simulink model "gm_combinedTxRx_AXIMM"  (R2017b)
settings: Solver=FixedStepDiscrete  StartTime=0.0  StopTime=10.0  RelTol=1e-3
InitFcn:
  | modelSettings
undefined symbols (not defined in the file or in its folder): coeff, filt, j, RadioSampleRate, VibertiTracebackLength, xPreambleSeq
libraries: hdlmdlgenlib x24, simulink x20, dsphdlfiltering x20, hdlsllib x10, dspsigops x5, commseqgen3 x4, commdigbbndpm3 x3, commcrc2 x2, commcnvcod2 x2, commsource2 x1, dspstat3 x1, dspmlti4 x1
(part 1 of 6)
settings Model: Creator=tcollins  LastModifiedBy=tcollins
settings OptimizationCC: BlockReduction=off  ConditionallyExecuteInputs=off  DefaultParameterBehavior=Inlined
settings DebuggingCC: AlgebraicLoopMsg=error  ArtificialAlgebraicLoopMsg=none  InheritedTsInSrcMsg=none  SingleTaskRateTransMsg=error  ParameterPrecisionLossMsg=none
settings HardwareCC: ProdBitPerPointer=32  ProdBitPerSizeT=32  ProdBitPerPtrDiffT=32  ProdLargestAtomicFloat=None  ProdIntDivRoundTo=Undefined  ProdEndianess=Unspecified  ProdWordSize=32  ProdHWDeviceType=ASIC/FPGA->ASIC/FPGA  ProdEqTarget=off
settings CodeAppCC: StateflowObjectComments=on

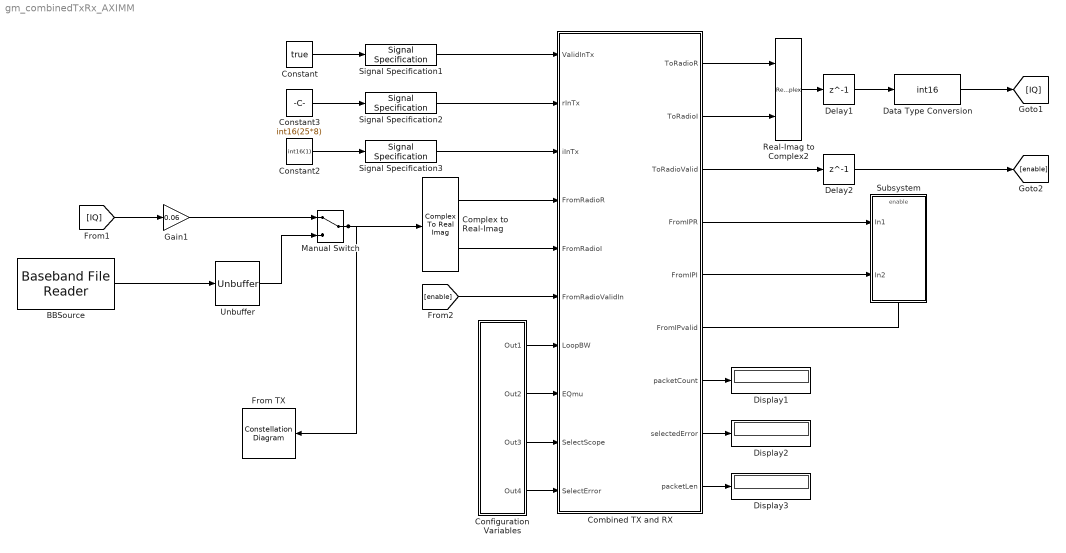
== system gm_combinedTxRx_AXIMM ==
  BBSource : commsource2/Baseband File Reader  Filename=PlutoCaptureQPSK.bb  InheritSampleTimeFromFile=off  SampleTime=100000/(RadioSampleRate)  SamplesPerFrame=100000  CyclicRepetition=off  FileEndOutputPort=off  SimulateUsing=Interpreted execution
      settings: SourceProductName=Communications System Toolbox  SourceProductBaseCode=CM
  Combined TX and RX : Subsystem  TreatAsAtomicUnit=on
  Complex to Real-Imag : ComplexToRealImag
  Configuration Variables : Subsystem
  Constant : Constant  Value=true  SampleTime=-1
  Constant2 : Constant  Value=int16(1)  SampleTime=-1
  Constant3 : Constant  Value=int16(25*8)  SampleTime=-1
  Data Type Conversion : DataTypeConversion  OutDataTypeStr=int16  ConvertRealWorld=Stored Integer (SI)
  Delay1 : Delay  DelayLength=1
  Delay2 : Delay  DelayLength=1
  Display1 : Display
  Display2 : Display
  Display3 : Display
  From TX : ConstellationDiagram
  Gain1 : Gain  Gain=0.06  OutDataTypeStr=int16
  Manual Switch : ManualSwitch
  Real-Imag to Complex2 : RealImagToComplex
  Signal Specification1 : SignalSpecification  OutDataTypeStr=boolean  SampleTime=1/RadioSampleRate
  Signal Specification2 : SignalSpecification  OutDataTypeStr=int16  SampleTime=1/RadioSampleRate
  Signal Specification3 : SignalSpecification  OutDataTypeStr=int16  SampleTime=1/RadioSampleRate
  Subsystem : Subsystem
  Unbuffer : Unbuffer
  wires:
  Configuration Variables/4(Out4) -> Combined TX and RX/10(SelectError)
  Combined TX and RX/9(packetLen) -> Display3/1
  Combined TX and RX/8(selectedError) -> Display2/1
  Combined TX and RX/7(packetCount) -> Display1/1
  Combined TX and RX/6(FromIPvalid) -> Subsystem/Enable
  Combined TX and RX/5(FromIPI) -> Subsystem/2(In2)
  Combined TX and RX/4(FromIPR) -> Subsystem/1(In1)
  Configuration Variables/3(Out3) -> Combined TX and RX/9(SelectScope)
  Configuration Variables/2(Out2) -> Combined TX and RX/8(EQmu)
  Configuration Variables/1(Out1) -> Combined TX and RX/7(LoopBW)
  Real-Imag to Complex2/1 -> Delay1/1
  Combined TX and RX/2(ToRadioI) -> Real-Imag to Complex2/2
  Combined TX and RX/1(ToRadioR) -> Real-Imag to Complex2/1
  Unbuffer/1 -> Manual Switch/2
  Complex to Real-Imag/2 -> Combined TX and RX/5(FromRadioI)
  Complex to Real-Imag/1 -> Combined TX and RX/4(FromRadioR)
  Gain1/1 -> Manual Switch/1
  [IQ] -> Gain1/1
  Signal Specification2/1 -> Combined TX and RX/2(rInTx)
  Manual Switch/1 -> Complex to Real-Imag/1, From TX/1
  Delay2/1 -> [enable]
  Data Type Conversion/1 -> [IQ]
  Delay1/1 -> Data Type Conversion/1
  Combined TX and RX/3(ToRadioValid) -> Delay2/1
  [enable] -> Combined TX and RX/6(FromRadioValidIn)
  Signal Specification3/1 -> Combined TX and RX/3(iInTx)
  Signal Specification1/1 -> Combined TX and RX/1(ValidInTx)
  BBSource/1 -> Unbuffer/1
  Constant/1 -> Signal Specification1/1
  Constant2/1 -> Signal Specification3/1
  Constant3/1 -> Signal Specification2/1

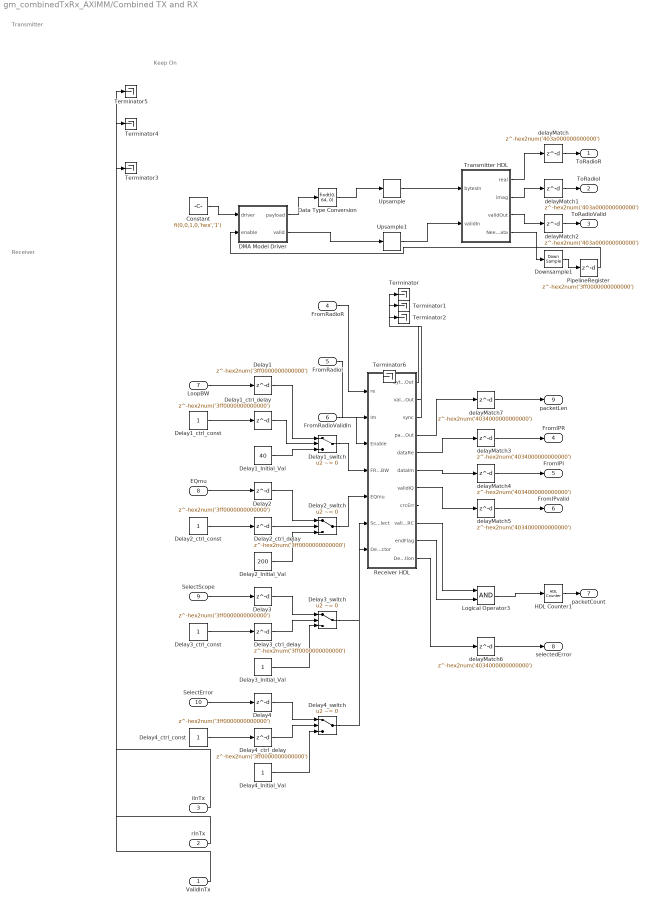
== system gm_combinedTxRx_AXIMM/Combined TX and RX ==
  note: Keep On
  note: Transmitter
  note: Receiver
  ValidInTx : Inport  OutDataTypeStr=boolean  SampleTime=1e-06
  rInTx : Inport  Port=2  OutDataTypeStr=int16  SampleTime=1e-06
  iInTx : Inport  Port=3  OutDataTypeStr=int16  SampleTime=1e-06
  FromRadioR : Inport  Port=4  OutDataTypeStr=int16  PortDimensions=1  SampleTime=1e-06
  FromRadioI : Inport  Port=5  OutDataTypeStr=int16  PortDimensions=1  SampleTime=1e-06
  FromRadioValidIn : Inport  Port=6  OutDataTypeStr=boolean  SampleTime=1e-06
  LoopBW : Inport  Port=7  OutDataTypeStr=int16  SampleTime=1e-06
  EQmu : Inport  Port=8  OutDataTypeStr=int16  SampleTime=1e-06
  SelectScope : Inport  Port=9  OutDataTypeStr=int8  SampleTime=1e-06
  SelectError : Inport  Port=10  OutDataTypeStr=int8  SampleTime=1e-06
  Constant : Constant  Value=fi(0,0,1,0,'hex','1')  OutDataTypeStr=boolean  SampleTime=-1
  DMA Model Driver : Subsystem
  Data Type Conversion : DataTypeConversion  OutDataTypeStr=fixdt(0, 64, 0)  SampleTime=4e-06
  Delay{1..4} (4 alike) : Delay  DelayLength=hex2num('3ff0000000000000')  InitialCondition=0  InputProcessing=Inherited  SampleTime=1e-06
  Delay1_Initial_Val : Constant  Value=40  OutDataTypeStr=int16  SampleTime=-1
  Delay1_ctrl_const : Constant  OutDataTypeStr=boolean  SampleTime=1e-06
  Delay1_ctrl_delay : Delay  DelayLength=hex2num('3ff0000000000000')  InitialCondition=0  InputProcessing=Inherited  SampleTime=1e-06
  Delay1_switch : Switch  Criteria=u2 ~= 0  Threshold=hex2num('0000000000000000')  OutDataTypeStr=int16  SampleTime=1e-06
  Delay2_Initial_Val : Constant  Value=200  OutDataTypeStr=int16  SampleTime=-1
  Delay2_ctrl_const : Constant  OutDataTypeStr=boolean  SampleTime=1e-06
  Delay2_ctrl_delay : Delay  DelayLength=hex2num('3ff0000000000000')  InitialCondition=0  InputProcessing=Inherited  SampleTime=1e-06
  Delay2_switch : Switch  Criteria=u2 ~= 0  Threshold=hex2num('0000000000000000')  OutDataTypeStr=int16  SampleTime=1e-06
  Delay3_Initial_Val : Constant  OutDataTypeStr=int8  SampleTime=-1
  Delay3_ctrl_const : Constant  OutDataTypeStr=boolean  SampleTime=1e-06
  Delay3_ctrl_delay : Delay  DelayLength=hex2num('3ff0000000000000')  InitialCondition=0  InputProcessing=Inherited  SampleTime=1e-06
  Delay3_switch : Switch  Criteria=u2 ~= 0  Threshold=hex2num('0000000000000000')  OutDataTypeStr=int8  SampleTime=1e-06
  Delay4_Initial_Val : Constant  OutDataTypeStr=int8  SampleTime=-1
  Delay4_ctrl_const : Constant  OutDataTypeStr=boolean  SampleTime=1e-06
  Delay4_ctrl_delay : Delay  DelayLength=hex2num('3ff0000000000000')  InitialCondition=0  InputProcessing=Inherited  SampleTime=1e-06
  Delay4_switch : Switch  Criteria=u2 ~= 0  Threshold=hex2num('0000000000000000')  OutDataTypeStr=int8  SampleTime=1e-06
  Downsample1 : DownSample  N=hex2num('4010000000000000')  phase=hex2num('0000000000000000')  RateOptions=Allow multirate processing
  HDL Counter1 : hdlsllib/Sources/HDL Counter  CountType=Count limited  CountInit=hex2num('0000000000000000')  CountStep=hex2num('3ff0000000000000')  CountMax=hex2num('41efffffffe00000')  CountFromType=Initial value  CountFrom=hex2num('0000000000000000')  CountResetPort=off  CountLoadPort=off  CountEnbPort=on  CountDirPort=off  CountDataType=Unsigned  CountWordLen=32  CountFracLen=0  CountSampTime=1e-06
      settings: SourceProductBaseCode=HD
  Logical Operator3 : Logic  AllPortsSameDT=off  OutDataTypeStr=boolean  SampleTime=1e-06
  PipelineRegister : Delay  DelayLength=hex2num('3ff0000000000000')  InitialCondition=0  InputProcessing=Inherited  SampleTime=4e-06
  Receiver HDL : Subsystem
      mask Display:
      | if ispc
      |     d = '\';
      | else
      |     d = '/';
      | end
      | model_path = get_param(bdroot, 'FileName');
      | %info = Simulink.MDLInfo(bdroot)
      | c = strsplit(model_path,d); c = strjoin(c(1:end-2),d);
      | logo = [c,d,'ADI_logo.svg'];
      | %disp(logo);
      | image(logo);
  Terminator{,1..6} (7 alike) : Terminator
  Transmitter HDL : Subsystem
      mask Display:
      | if ispc
      |     d = '\';
      | else
      |     d = '/';
      | end
      | model_path = get_param(bdroot, 'FileName');
      | %info = Simulink.MDLInfo(bdroot)
      | c = strsplit(model_path,d); c = strjoin(c(1:end-2),d);
      | logo = [c,d,'ADI_logo.svg'];
      | %disp(logo);
      | image(logo);
  Upsample : dspsigops/Upsample  N=hex2num('4010000000000000')  phase=hex2num('0000000000000000')  RateOptions=Allow multirate processing  ic=0  mode=Unused parameter value
  Upsample1 : dspsigops/Upsample  N=hex2num('4010000000000000')  phase=hex2num('0000000000000000')  RateOptions=Allow multirate processing  ic=0  mode=Unused parameter value
  delayMatch : Delay  DelayLength=hex2num('403a000000000000')  InitialCondition=0  InputProcessing=Inherited  SampleTime=1e-06
  delayMatch1 : Delay  DelayLength=hex2num('403a000000000000')  InitialCondition=0  InputProcessing=Inherited  SampleTime=1e-06
  delayMatch2 : Delay  DelayLength=hex2num('403a000000000000')  InitialCondition=0  InputProcessing=Inherited  SampleTime=1e-06
  delayMatch{3..7} (5 alike) : Delay  DelayLength=hex2num('4034000000000000')  InitialCondition=0  InputProcessing=Inherited  SampleTime=1e-06
  ToRadioR : Outport
  ToRadioI : Outport  Port=2
  ToRadioValid : Outport  Port=3
  FromIPR : Outport  Port=4
  FromIPI : Outport  Port=5
  FromIPvalid : Outport  Port=6
  packetCount : Outport  Port=7
  selectedError : Outport  Port=8
  packetLen : Outport  Port=9
  wires:
  ValidInTx/1 -> Terminator5/1
  rInTx/1 -> Terminator4/1
  iInTx/1 -> Terminator3/1
  FromRadioR/1 -> Receiver HDL/1(re)
  FromRadioI/1 -> Receiver HDL/2(Im)
  FromRadioValidIn/1 -> Receiver HDL/3(Enable)
  LoopBW/1 -> Delay1/1
  EQmu/1 -> Delay2/1
  SelectScope/1 -> Delay3/1
  SelectError/1 -> Delay4/1
  Delay1_switch/1 -> Receiver HDL/4(FRLoopBW)
  Delay2_switch/1 -> Receiver HDL/5(EQmu)
  Delay3_switch/1 -> Receiver HDL/6(Scope Select)
  Delay4_switch/1 -> Receiver HDL/7(DebugSelector)
  HDL Counter1/1 -> packetCount/1
  Logical Operator3/1 -> HDL Counter1/1
  Receiver HDL/1(bytesOut) -> Terminator/1
  Receiver HDL/2(validOut) -> Terminator1/1
  Receiver HDL/3(sync) -> Terminator2/1
  delayMatch7/1 -> packetLen/1
  delayMatch3/1 -> FromIPR/1
  delayMatch4/1 -> FromIPI/1
  delayMatch5/1 -> FromIPvalid/1
  Receiver HDL/8(crcErr) -> Terminator6/1
  Receiver HDL/9(validCRC) -> Logical Operator3/1
  Receiver HDL/10(endFlag) -> Logical Operator3/2
  delayMatch6/1 -> selectedError/1
  delayMatch/1 -> ToRadioR/1
  delayMatch1/1 -> ToRadioI/1
  delayMatch2/1 -> ToRadioValid/1
  Delay1/1 -> Delay1_switch/1
  Delay1_ctrl_const/1 -> Delay1_ctrl_delay/1
  Delay1_ctrl_delay/1 -> Delay1_switch/2
  Delay2/1 -> Delay2_switch/1
  Delay2_ctrl_const/1 -> Delay2_ctrl_delay/1
  Delay2_ctrl_delay/1 -> Delay2_switch/2
  Delay3/1 -> Delay3_switch/1
  Delay3_ctrl_const/1 -> Delay3_ctrl_delay/1
  Delay3_ctrl_delay/1 -> Delay3_switch/2
  Delay4/1 -> Delay4_switch/1
  Delay4_ctrl_const/1 -> Delay4_ctrl_delay/1
  Delay4_ctrl_delay/1 -> Delay4_switch/2
  Constant/1 -> DMA Model Driver/1(driver)
  Delay1_Initial_Val/1 -> Delay1_switch/3
  Delay2_Initial_Val/1 -> Delay2_switch/3
  Delay3_Initial_Val/1 -> Delay3_switch/3
  Delay4_Initial_Val/1 -> Delay4_switch/3
  Transmitter HDL/1(real) -> delayMatch/1
  Transmitter HDL/2(imag) -> delayMatch1/1
  Transmitter HDL/3(validOut) -> delayMatch2/1
  Receiver HDL/5(dataRe) -> delayMatch3/1
  Receiver HDL/6(dataIm) -> delayMatch4/1
  Receiver HDL/7(validIQ) -> delayMatch5/1
  Receiver HDL/11(DebugSelection) -> delayMatch6/1
  Receiver HDL/4(payloadLenOut) -> delayMatch7/1
  Upsample1/1 -> Transmitter HDL/2(validIn)
  PipelineRegister/1 -> DMA Model Driver/2(enable)
  DMA Model Driver/1(payload) -> Data Type Conversion/1
  DMA Model Driver/2(valid) -> Upsample1/1
  Data Type Conversion/1 -> Upsample/1
  Upsample/1 -> Transmitter HDL/1(bytesIn)
  Transmitter HDL/4(Need Data) -> Downsample1/1
  Downsample1/1 -> PipelineRegister/1

== system gm_combinedTxRx_AXIMM/Configuration Variables ==
  1/mu : Constant  Value=200  OutDataTypeStr=int16  SampleTime=-1
  Constant4 : Constant  Value=int8(3)  SampleTime=1/RadioSampleRate
  Error Status Selector : Constant  Value=int8(4)  SampleTime=1/RadioSampleRate
  Index of LBW Lookup : Constant  Value=int16(40)  SampleTime=1/RadioSampleRate
  Out1 : Outport
  Out2 : Outport  Port=2
  Out3 : Outport  Port=3
  Out4 : Outport  Port=4
  wires:
  Error Status Selector/1 -> Out4/1
  Constant4/1 -> Out3/1
  Index of LBW Lookup/1 -> Out1/1
  1/mu/1 -> Out2/1

== system gm_combinedTxRx_AXIMM/Subsystem ==
  In1 : Inport
  In2 : Inport  Port=2
  Enable : EnablePort
  Real-Imag to Complex : RealImagToComplex
  Selected IQ : ConstellationDiagram
  wires:
  Real-Imag to Complex/1 -> Selected IQ/1
  In1/1 -> Real-Imag to Complex/1
  In2/1 -> Real-Imag to Complex/2

== system gm_combinedTxRx_AXIMM/Combined TX and RX/DMA Model Driver ==
  driver : Inport  SampleTime=4e-06
  enable : Inport  Port=2  SampleTime=4e-06
  DMA Model Driver : MATLAB Function  TreatAsAtomicUnit=on
  payload : Outport
  valid : Outport  Port=2
  wires:
  driver/1 -> DMA Model Driver/1(driver)
  enable/1 -> DMA Model Driver/2(enable)
  DMA Model Driver/1(payload) -> payload/1
  DMA Model Driver/2(valid) -> valid/1

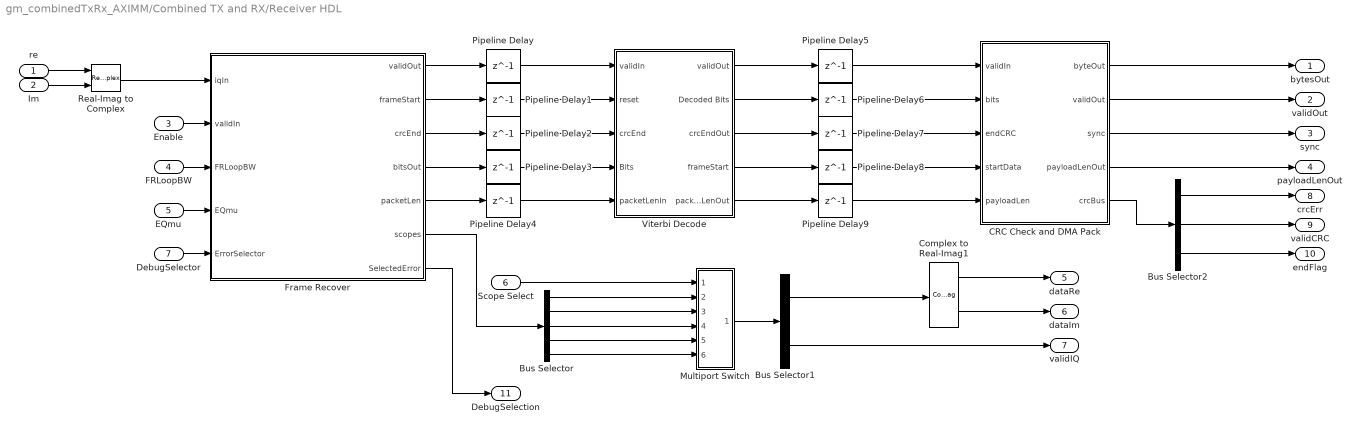
== system gm_combinedTxRx_AXIMM/Combined TX and RX/Receiver HDL ==
  re : Inport  OutDataTypeStr=int16  SampleTime=1e-06
  Im : Inport  Port=2  OutDataTypeStr=int16  SampleTime=1e-06
  Enable : Inport  Port=3  OutDataTypeStr=boolean  SampleTime=1e-06
  FRLoopBW : Inport  Port=4  OutDataTypeStr=int16  SampleTime=1e-06
  EQmu : Inport  Port=5  OutDataTypeStr=int16  SampleTime=1e-06
  Scope Select : Inport  Port=6  OutDataTypeStr=int8  SampleTime=1e-06
  DebugSelector : Inport  Port=7  OutDataTypeStr=int8  SampleTime=1e-06
  Bus Selector : BusSelector  OutputSignals=After SRRC,After Timing,After Frequency,After EQ,From Radio
  Bus Selector1 : BusSelector  OutputSignals=signal1,signal2
  Bus Selector2 : BusSelector  OutputSignals=err,valid,end
  CRC Check and DMA Pack : Subsystem
  Complex to Real-Imag1 : ComplexToRealImag
  Frame Recover : Subsystem
  Multiport Switch : Subsystem
  Pipeline Delay{,1..9} (10 alike) : Delay  DelayLength=1
  Real-Imag to Complex : RealImagToComplex
  Viterbi Decode : Subsystem
  bytesOut : Outport
  validOut : Outport  Port=2
  sync : Outport  Port=3
  payloadLenOut : Outport  Port=4
  dataRe : Outport  Port=5
  dataIm : Outport  Port=6
  validIQ : Outport  Port=7
  crcErr : Outport  Port=8
  validCRC : Outport  Port=9
  endFlag : Outport  Port=10
  DebugSelection : Outport  Port=11
  wires:
  Bus Selector/1 -> Multiport Switch/2(Multiport Switch_In2)
  Bus Selector/2 -> Multiport Switch/3(Multiport Switch_In3)
  Bus Selector/3 -> Multiport Switch/4(Multiport Switch_In4)
  Bus Selector/4 -> Multiport Switch/5(Multiport Switch_In5)
  Bus Selector/5 -> Multiport Switch/6(Multiport Switch_In6)
  Bus Selector1/1 -> Complex to Real-Imag1/1
  Bus Selector1/2 -> validIQ/1
  Bus Selector2/1 -> crcErr/1
  Bus Selector2/2 -> validCRC/1
  Bus Selector2/3 -> endFlag/1
  CRC Check and DMA Pack/1(byteOut) -> bytesOut/1
  CRC Check and DMA Pack/2(validOut) -> validOut/1
  CRC Check and DMA Pack/3(sync) -> sync/1
  CRC Check and DMA Pack/4(payloadLenOut) -> payloadLenOut/1
  CRC Check and DMA Pack/5(crcBus) -> Bus Selector2/1
  Complex to Real-Imag1/1 -> dataRe/1
  Complex to Real-Imag1/2 -> dataIm/1
  Frame Recover/1(validOut) -> Pipeline Delay/1
  Frame Recover/2(frameStart) -> Pipeline Delay1/1
  Frame Recover/3(crcEnd) -> Pipeline Delay2/1
  Frame Recover/4(bitsOut) -> Pipeline Delay3/1
  Frame Recover/5(packetLen) -> Pipeline Delay4/1
  Frame Recover/6(scopes) -> Bus Selector/1
  Frame Recover/7(SelectedError) -> DebugSelection/1
  Multiport Switch/1(Multiport Switch_Out1) -> Bus Selector1/1
  Pipeline Delay/1 -> Viterbi Decode/1(validIn)
  Pipeline Delay1/1 -> Viterbi Decode/2(reset)
  Pipeline Delay2/1 -> Viterbi Decode/3(crcEnd)
  Pipeline Delay3/1 -> Viterbi Decode/4(Bits)
  Pipeline Delay4/1 -> Viterbi Decode/5(packetLenIn)
  Pipeline Delay5/1 -> CRC Check and DMA Pack/1(validIn)
  Pipeline Delay6/1 -> CRC Check and DMA Pack/2(bits)
  Pipeline Delay7/1 -> CRC Check and DMA Pack/3(endCRC)
  Pipeline Delay8/1 -> CRC Check and DMA Pack/4(startData)
  Pipeline Delay9/1 -> CRC Check and DMA Pack/5(payloadLen)
  Real-Imag to Complex/1 -> Frame Recover/1(iqIn)
  Viterbi Decode/1(validOut) -> Pipeline Delay5/1
  Viterbi Decode/2(Decoded Bits) -> Pipeline Delay6/1
  Viterbi Decode/3(crcEndOut) -> Pipeline Delay7/1
  Viterbi Decode/4(frameStart) -> Pipeline Delay8/1
  Viterbi Decode/5(packetLenOut) -> Pipeline Delay9/1
  re/1 -> Real-Imag to Complex/1
  Im/1 -> Real-Imag to Complex/2
  Enable/1 -> Frame Recover/2(validIn)
  FRLoopBW/1 -> Frame Recover/3(FRLoopBW)
  EQmu/1 -> Frame Recover/4(EQmu)
  Scope Select/1 -> Multiport Switch/1(Multiport Switch_In1)
  DebugSelector/1 -> Frame Recover/5(ErrorSelector)

== system gm_combinedTxRx_AXIMM/Combined TX and RX/Transmitter HDL ==
  bytesIn : Inport  OutDataTypeStr=fixdt(0, 64, 0)  SampleTime=1e-06
  validIn : Inport  Port=2  OutDataTypeStr=boolean  SampleTime=1e-06
  Complex to Real-Imag : ComplexToRealImag  SampleTime=1e-06
  DMA Interface : Subsystem
  Delay : Delay  DelayLength=hex2num('3ff0000000000000')  InitialCondition=0  InputProcessing=Inherited  SampleTime=4e-06
  Display : Display
  Keep Transmitting Always : Constant  Value=fi(0,0,1,0,'hex','1')  OutDataTypeStr=boolean  SampleTime=-1
  Keep Transmitting Always_out1_wire : dspsigops/Repeat  N=hex2num('4010000000000000')  RateOptions=Allow multirate processing  ic=0  mode=Unused parameter value
      settings: SourceProductName=DSP System Toolbox
  Packet Generation : Subsystem
  Raised Cosine Transmit Filter1 : Subsystem  mask(Raised Cosine Transmit Filter){filtType=Square root, R=hex2num('3fe0000000000000'), filtSpan=hex2num('4020000000000000'), N=hex2num('4010000000000000'), filterGain=hex2num('3ff0000000000000'), InputProcessing=Elements as channels (sample based), RateOptions=Allow multirate processing, framing=Mute, checkCoeff=off, variableName=rcTxFilt1, checkGain=Normalized, sampMode=Mute, saveAsFlag=hex2num('0000000000000000'), currentFiltSpan=hex2num('4020000000000000'), D=hex2num('4010000000000000'), launchFVT=on, roundingMode=Floor, overflowMode=off, coeffMode=Same word length as input, coeffWordLength=hex2num('4030000000000000'), coeffFracLength=hex2num('402e000000000000'), coeffDataTypeStr=Inherit: Same word length as input, coeffMin=[], coeffMax=[], coeffLastDataTypeStr=Inherit: Same word length as input, prodOutputMode=Inherit via internal rule, prodOutputWordLength=hex2num('4040000000000000'), prodOutputFracLength=hex2num('403e000000000000'), prodOutputDataTypeStr=Inherit: Inherit via internal rule, prodOutputLastDataTypeStr=Inherit: Inherit via internal rule, accumMode=Inherit via internal rule, accumWordLength=hex2num('4040000000000000'), accumFracLength=hex2num('403e000000000000'), accumDataTypeStr=Inherit: Inherit via internal rule, accumLastDataTypeStr=Inherit: Inherit via internal rule, outputMode=Binary point scaling, outputWordLength=hex2num('4030000000000000'), outputFracLength=hex2num('402c000000000000'), outputDataTypeStr=fixdt(1,hex2num('4030000000000000'),hex2num('402c000000000000')), outputMin=[], outputMax=[], outputLastDataTypeStr=fixdt(1,hex2num('4030000000000000'),hex2num('402c000000000000')), LockScale=off}
      mask prompts: filtType "Filter shape:"; R "Rolloff factor:"; filtSpan "Filter span in symbols:"; N "Output samples per symbol:"; filterGain "Linear amplitude filter gain:"; InputProcessing "dsp:FIRMultirateBlockDialog:InputProc_MP"; RateOptions "dsp:FIRMultirateBlockDialog:RateOptions_MP"; checkCoeff "Export filter coefficients to workspace"; variableName "Coefficient variable name:"; checkGain "Filter gain:"; sampMode "Input sampling mode:"; saveAsFlag "Save_as flag:"; currentFiltSpan "Current filter span in symbols:"; D "Group delay (number of symbols):"; launchFVT "Visualize filter with FVTool"; roundingMode "dspshared:FixptDialog:roundingMode"; overflowMode "Simulink:masks:SaturateOnIntegerOverflow_MP"; LockScale "dspshared:FixptDialog:lockAgnstChanges"
      mask help: Upsample and filter the input signal using a normal or square root raised cosine FIR filter.
      mask init:
      | commblkrcfilttx(gcbh,'frameupgrademultirate');
      | 
      | [filt, icon, err] = commblkrcfilttx(gcbh,'init',...
      |     filtType, R, filtSpan, currentFiltSpan, D, N, filterGain, ...
      |     checkCoeff, variableName);
      | 
      | % Set sample modes of underlying blocks
      | commblkrcfilttx(gcb,'setFIRInterp', InputProcessing, RateOptions, ...
      |     roundingMode, overflowMode, LockScale);
      | 
      | if(~isempty(err.msg))
      | 	error(err.eID,err.msg);
      | end
      mask Help: eval('blocksethelp');
      mask TypeOptions filtType: Normal | Square root
      mask TypeOptions InputProcessing: Columns as channels (frame based) | Elements as channels (sample based)
      mask Callback InputProcessing: commblkrcfilttx(gcbh,'cbInputProcessing');
      mask TypeOptions RateOptions: Enforce single-rate processing | Allow multirate processing
      mask TypeOptions framing: Enforce single-rate processing | Allow multirate processing | Maintain input frame rate | Maintain input frame size | Mute
      mask Callback checkCoeff: commblkrcfilttx(gcbh,'cbCheckCoeff');
      mask Callback variableName: commblkrcfilttx(gcbh,'dialogdynamic');
      mask TypeOptions checkGain: Normalized | User-specified
      mask TypeOptions sampMode: Frame-based | Sample-based | Mute
      mask TypeOptions roundingMode: Ceiling | Convergent | Floor | Nearest | Round | Simplest | Zero
      mask TypeOptions coeffMode: Same word length as input | Specify word length | Binary point scaling | Slope and bias scaling
      mask TypeOptions prodOutputMode: Inherit via internal rule | Same as input | Binary point scaling | Slope and bias scaling
      mask TypeOptions accumMode: Inherit via internal rule | Same as product output | Same as input | Binary point scaling | Slope and bias scaling
      mask TypeOptions outputMode: Same as accumulator | Same as product output | Same as input | Binary point scaling | Slope and bias scaling
      mask Display:
      | plot(0,0,1,1,icon.xx,icon.plot);
      | text(icon.x,icon.y,icon.str,'horiz','center');
  Subsystem : Subsystem
  Subsystem1 : Subsystem
  Terminator : Terminator
  Terminator1 : Terminator
  Transmit Constellation Diagram : ConstellationDiagram
  readyForInput_wire : dspsigops/Repeat  N=hex2num('4010000000000000')  RateOptions=Allow multirate processing  ic=0  mode=Unused parameter value
      settings: SourceProductName=DSP System Toolbox
  real : Outport
  imag : Outport  Port=2
  validOut : Outport  Port=3
  Need Data : Outport  Port=4
  wires:
  bytesIn/1 -> Subsystem/1(In1)
  validIn/1 -> Subsystem1/1(In1)
  Complex to Real-Imag/1 -> real/1
  Complex to Real-Imag/2 -> imag/1
  DMA Interface/1(validOut) -> Terminator1/1
  DMA Interface/2(bit) -> Packet Generation/1(bits)
  DMA Interface/3(payloadLength) -> Packet Generation/2(payloadSize)
  DMA Interface/4(startOut) -> Packet Generation/3(start)
  DMA Interface/5(readyForMore) -> readyForInput_wire/1
  Delay/1 -> DMA Interface/3(EOF)
  Keep Transmitting Always/1 -> Keep Transmitting Always_out1_wire/1
  Packet Generation/1(trueData) -> Terminator/1
  Packet Generation/2(symbols) -> Raised Cosine Transmit Filter1/1(In1)
  Packet Generation/3(EOF) -> Delay/1
  Raised Cosine Transmit Filter1/1(Out1) -> Complex to Real-Imag/1, Transmit Constellation Diagram/1
  Keep Transmitting Always_out1_wire/1 -> Display/1, validOut/1
  readyForInput_wire/1 -> Need Data/1
  Subsystem/1(Out1) -> DMA Interface/1(byteIn)
  Subsystem1/1(Out1) -> DMA Interface/2(validIn)

== system gm_combinedTxRx_AXIMM/Combined TX and RX/Receiver HDL/CRC Check and DMA Pack ==
  validIn : Inport  PortDimensions=1  SampleTime=1e-06
  bits : Inport  Port=2  PortDimensions=1  SampleTime=1e-06
  endCRC : Inport  Port=3  PortDimensions=1  SampleTime=1e-06
  startData : Inport  Port=4  PortDimensions=1  SampleTime=1e-06
  payloadLen : Inport  Port=5  PortDimensions=1  SampleTime=1e-06
  Bus Creator : BusCreator  Inputs=3
  CRC Check ES : Subsystem
  DMA Interface : Subsystem
  Pipeline Delay{,1..5} (6 alike) : Delay  DelayLength=1
  byteOut : Outport
  validOut : Outport  Port=2
  sync : Outport  Port=3
  payloadLenOut : Outport  Port=4
  crcBus : Outport  Port=5
  wires:
  Bus Creator/1 -> crcBus/1
  CRC Check ES/1(dataOut) -> Pipeline Delay/1
  CRC Check ES/2(startOut) -> Pipeline Delay1/1
  CRC Check ES/3(endOut) -> Pipeline Delay2/1
  CRC Check ES/4(validOut) -> Pipeline Delay3/1
  CRC Check ES/5(err) -> Pipeline Delay4/1
  CRC Check ES/6(payloadLenOut) -> Pipeline Delay5/1
  DMA Interface/1(byteOut) -> byteOut/1
  DMA Interface/2(validOut) -> validOut/1
  DMA Interface/3(sync) -> sync/1
  DMA Interface/4(payloadLenOut) -> payloadLenOut/1
  Pipeline Delay/1 -> DMA Interface/1(bitIn)
  Pipeline Delay1/1 -> DMA Interface/2(startIn)
  Pipeline Delay2/1 -> Bus Creator/3, DMA Interface/3(endIn)  "end"
  Pipeline Delay3/1 -> Bus Creator/2, DMA Interface/4(validIn)  "valid"
  Pipeline Delay4/1 -> Bus Creator/1, DMA Interface/5(err)  "err"
  Pipeline Delay5/1 -> DMA Interface/6(payloadLen)
  validIn/1 -> CRC Check ES/1(Valid)
  bits/1 -> CRC Check ES/2(Bits)
  endCRC/1 -> CRC Check ES/3(endCRC)
  startData/1 -> CRC Check ES/4(StartData)
  payloadLen/1 -> CRC Check ES/5(payloadLen)

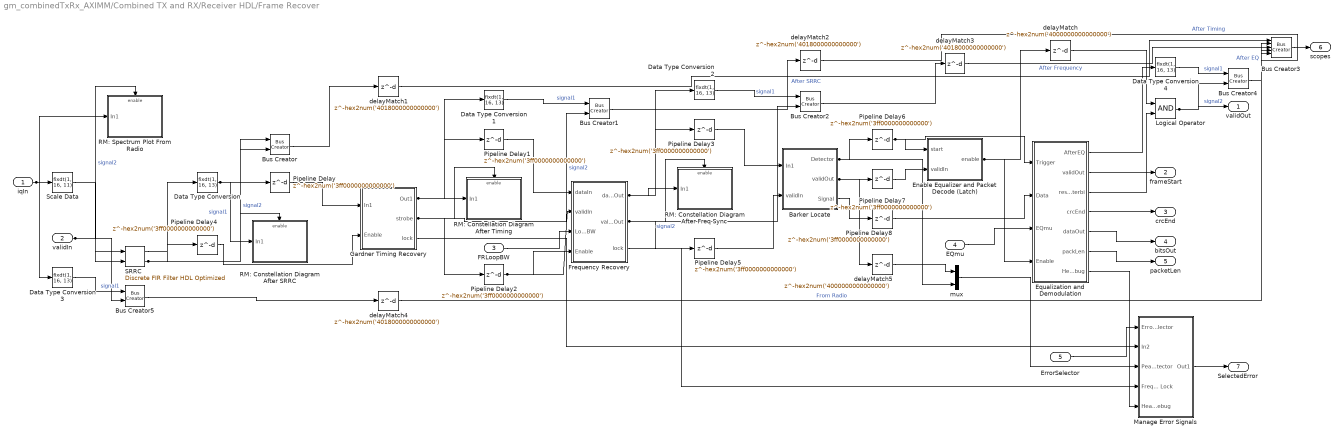
== system gm_combinedTxRx_AXIMM/Combined TX and RX/Receiver HDL/Frame Recover ==
  iqIn : Inport  PortDimensions=1  SampleTime=1e-06
  validIn : Inport  Port=2  PortDimensions=1  SampleTime=1e-06
  FRLoopBW : Inport  Port=3  SampleTime=1e-06
  EQmu : Inport  Port=4  SampleTime=1e-06
  ErrorSelector : Inport  Port=5  PortDimensions=1  SampleTime=1e-06
  Barker Locate : Subsystem  mask{Threshold=hex2num('3ff0000000000000')}
  Bus Creator{,1..2,4..5} (5 alike) : BusCreator  Inputs=2
  Bus Creator3 : BusCreator  Inputs=5
  Data Type Conversion{,1..4} (5 alike) : DataTypeConversion  OutDataTypeStr=fixdt(1, 16, 13)  SampleTime=1e-06
  Enable Equalizer and Packet Decode (Latch) : Subsystem
  Equalization and Demodulation : Subsystem
  Frequency Recovery : Subsystem
  Gardner Timing Recovery : Subsystem
  Logical Operator : Logic  AllPortsSameDT=off  OutDataTypeStr=boolean  SampleTime=1e-06
  Manage Error Signals : Subsystem
  Pipeline Delay{,1..8} (9 alike) : Delay  DelayLength=hex2num('3ff0000000000000')  InitialCondition=0  InputProcessing=Inherited  SampleTime=1e-06
  RM: Constellation Diagram After Freq Sync : Subsystem
  RM: Constellation Diagram After SRRC : Subsystem
  RM: Constellation Diagram After Timing : Subsystem
  RM: Spectrum Plot From Radio : Subsystem
  SRRC : dsphdlfiltering/Discrete FIR Filter HDL Optimized  Numerator=coeff  Sharing=off  SharingFactor=2  SimulateUsing=Code generation  roundingMode=Floor  overflowMode=on  CoefficientsDataTypeStr=Inherit: Same word length as input  CoefficientsMin=[]  CoefficientsMax=[]  OutputDataTypeStr=fixdt(1,16,11)  OutputMin=[]  OutputMax=[]  ValidInPort=on  ReadyPort=off
      settings: SourceProductName=DSP System Toolbox  SourceProductBaseCode=DS
  Scale Data : DataTypeConversion  OutDataTypeStr=fixdt(1, 16, 11)  ConvertRealWorld=Stored Integer (SI)  SampleTime=1e-06  SaturateOnIntegerOverflow=on
  delayMatch : Delay  DelayLength=hex2num('4000000000000000')  InitialCondition=0  InputProcessing=Inherited  SampleTime=1e-06
  delayMatch{1..4} (4 alike) : Delay  DelayLength=hex2num('4018000000000000')  InitialCondition=0  InputProcessing=Inherited  SampleTime=1e-06
  delayMatch5 : Delay  DelayLength=hex2num('4000000000000000')  InitialCondition=0  InputProcessing=Inherited  SampleTime=1e-06
  mux : Mux  Inputs=2
  validOut : Outport
  frameStart : Outport  Port=2
  crcEnd : Outport  Port=3
  bitsOut : Outport  Port=4
  packetLen : Outport  Port=5
  scopes : Outport  Port=6
  SelectedError : Outport  Port=7
  wires:
  Barker Locate/1(Detector) -> mux/2, Pipeline Delay6/1
  delayMatch5/1 -> mux/1
  Barker Locate/3(Signal) -> Pipeline Delay8/1
  delayMatch1/1 -> Bus Creator3/1  "After SRRC"
  delayMatch2/1 -> Bus Creator3/2  "After Timing"
  delayMatch3/1 -> Bus Creator3/3  "After Frequency"
  Bus Creator3/1 -> scopes/1
  Bus Creator4/1 -> Bus Creator3/4  "After EQ"
  delayMatch4/1 -> Bus Creator3/5  "From Radio"
  Data Type Conversion/1 -> Bus Creator/1, Pipeline Delay/1, RM: Constellation Diagram After SRRC/1(In1)  "signal1"
  Data Type Conversion1/1 -> Bus Creator1/1  "signal1"
  Data Type Conversion2/1 -> Bus Creator2/1  "signal1"
  Data Type Conversion3/1 -> Bus Creator5/1  "signal1"
  Data Type Conversion4/1 -> Bus Creator4/1  "signal1"
  delayMatch/1 -> Logical Operator/1
  Equalization and Demodulation/1(AfterEQ) -> Data Type Conversion4/1
  Equalization and Demodulation/2(validOut) -> Logical Operator/2
  Equalization and Demodulation/3(resetViterbi) -> frameStart/1
  Equalization and Demodulation/4(crcEnd) -> crcEnd/1
  Equalization and Demodulation/5(dataOut) -> bitsOut/1
  Equalization and Demodulation/6(packLen) -> packetLen/1
  Equalization and Demodulation/7(HeaderDebug) -> Manage Error Signals/5(Header Debug)
  Frequency Recovery/1(dataOut) -> Data Type Conversion2/1, Pipeline Delay3/1, RM: Constellation Diagram After Freq Sync/1(In1)
  Frequency Recovery/2(validOut) -> Bus Creator2/2, Pipeline Delay5/1, RM: Constellation Diagram After Freq Sync/Enable  "signal2"
  Frequency Recovery/3(lock) -> Manage Error Signals/4(FreqPLL Lock)
  Gardner Timing Recovery/1(Out1) -> Data Type Conversion1/1, Pipeline Delay1/1, RM: Constellation Diagram After Timing/1(In1)
  Gardner Timing Recovery/2(strobe) -> Bus Creator1/2, Pipeline Delay2/1, RM: Constellation Diagram After Timing/Enable  "signal2"
  Gardner Timing Recovery/3(lock) -> Manage Error Signals/2(In2)
  Logical Operator/1 -> Bus Creator4/2, validOut/1  "signal2"
  Manage Error Signals/1(Out1) -> SelectedError/1
  mux/1 -> Manage Error Signals/3(Peak Detector)
  Pipeline Delay/1 -> Gardner Timing Recovery/1(In1)
  Pipeline Delay1/1 -> Frequency Recovery/1(dataIn)
  Pipeline Delay2/1 -> Frequency Recovery/2(validIn), Frequency Recovery/4(Enable)
  Pipeline Delay3/1 -> Barker Locate/1(In1)
  Pipeline Delay4/1 -> Gardner Timing Recovery/2(Enable)
  Pipeline Delay5/1 -> Barker Locate/2(validIn)
  Pipeline Delay6/1 -> Enable Equalizer and Packet Decode (Latch)/1(start), Equalization and Demodulation/1(Trigger)
  Pipeline Delay7/1 -> Enable Equalizer and Packet Decode (Latch)/2(validIn)
  Pipeline Delay8/1 -> Equalization and Demodulation/2(Data)
  SRRC/1 -> Data Type Conversion/1
  SRRC/2 -> Bus Creator/2, Pipeline Delay4/1, RM: Constellation Diagram After SRRC/Enable  "signal2"
  Scale Data/1 -> SRRC/1
  iqIn/1 -> Scale Data/1, Data Type Conversion3/1, RM: Spectrum Plot From Radio/1(In1)
  validIn/1 -> Bus Creator5/2, RM: Spectrum Plot From Radio/Enable, SRRC/2  "signal2"
  FRLoopBW/1 -> Frequency Recovery/3(LoopBW)
  EQmu/1 -> Equalization and Demodulation/3(EQmu)
  ErrorSelector/1 -> Manage Error Signals/1(ErrorSelector)
  Enable Equalizer and Packet Decode (Latch)/1(enable) -> delayMatch/1, Equalization and Demodulation/4(Enable)
  Bus Creator/1 -> delayMatch1/1
  Bus Creator1/1 -> delayMatch2/1
  Bus Creator2/1 -> delayMatch3/1
  Bus Creator5/1 -> delayMatch4/1
  Barker Locate/2(validOut) -> delayMatch5/1, Pipeline Delay7/1

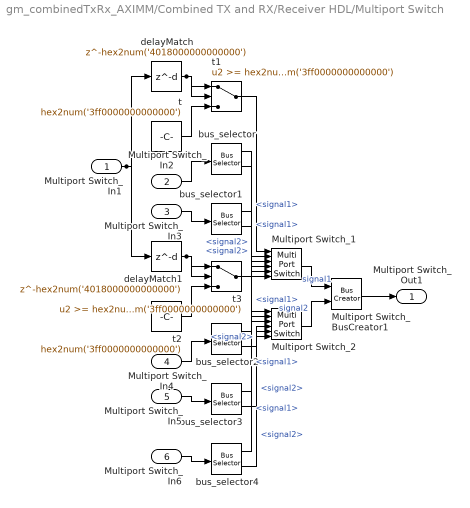
== system gm_combinedTxRx_AXIMM/Combined TX and RX/Receiver HDL/Multiport Switch ==
  Multiport Switch_In1 : Inport  SampleTime=1e-06
  Multiport Switch_In2 : Inport  Port=2  SampleTime=1e-06
  Multiport Switch_In3 : Inport  Port=3  SampleTime=1e-06
  Multiport Switch_In4 : Inport  Port=4  SampleTime=1e-06
  Multiport Switch_In5 : Inport  Port=5  SampleTime=1e-06
  Multiport Switch_In6 : Inport  Port=6  SampleTime=1e-06
  Multiport Switch_1 : MultiPortSwitch  Inputs=5  DiagnosticForDefault=None  OutDataTypeStr=fixdt(1, 16, 13)  SampleTime=1e-06
  Multiport Switch_2 : MultiPortSwitch  Inputs=5  DiagnosticForDefault=None  SampleTime=1e-06
  Multiport Switch_BusCreator1 : BusCreator  Inputs=2
  bus_selector{,1..4} (5 alike) : BusSelector  OutputSignals=signal1,signal2
  delayMatch : Delay  DelayLength=hex2num('4018000000000000')  InitialCondition=0  InputProcessing=Inherited  SampleTime=1e-06
  delayMatch1 : Delay  DelayLength=hex2num('4018000000000000')  InitialCondition=0  InputProcessing=Inherited  SampleTime=1e-06
  t : Constant  Value=hex2num('3ff0000000000000')  OutDataTypeStr=int8  SampleTime=-1
  t1 : Switch  Threshold=hex2num('3ff0000000000000')  OutDataTypeStr=int8  SampleTime=1e-06
  t2 : Constant  Value=hex2num('3ff0000000000000')  OutDataTypeStr=int8  SampleTime=-1
  t3 : Switch  Threshold=hex2num('3ff0000000000000')  OutDataTypeStr=int8  SampleTime=1e-06
  Multiport Switch_Out1 : Outport
  wires:
  delayMatch/1 -> t1/2, t1/1
  Multiport Switch_1/1 -> Multiport Switch_BusCreator1/1  "signal1"
  Multiport Switch_2/1 -> Multiport Switch_BusCreator1/2  "signal2"
  Multiport Switch_BusCreator1/1 -> Multiport Switch_Out1/1
  bus_selector/1 -> Multiport Switch_1/2  "<signal1>"
  bus_selector/2 -> Multiport Switch_2/2  "<signal2>"
  bus_selector1/1 -> Multiport Switch_1/3  "<signal1>"
  bus_selector1/2 -> Multiport Switch_2/3  "<signal2>"
  bus_selector2/1 -> Multiport Switch_1/4  "<signal1>"
  bus_selector2/2 -> Multiport Switch_2/4  "<signal2>"
  bus_selector3/1 -> Multiport Switch_1/5  "<signal1>"
  bus_selector3/2 -> Multiport Switch_2/5  "<signal2>"
  bus_selector4/1 -> Multiport Switch_1/6  "<signal1>"
  bus_selector4/2 -> Multiport Switch_2/6  "<signal2>"
  Multiport Switch_In1/1 -> delayMatch1/1, delayMatch/1
  Multiport Switch_In2/1 -> bus_selector/1
  Multiport Switch_In3/1 -> bus_selector1/1
  Multiport Switch_In4/1 -> bus_selector2/1
  Multiport Switch_In5/1 -> bus_selector3/1
  Multiport Switch_In6/1 -> bus_selector4/1
  delayMatch1/1 -> t3/2, t3/1
  t/1 -> t1/3
  t1/1 -> Multiport Switch_1/1
  t2/1 -> t3/3
  t3/1 -> Multiport Switch_2/1

== system gm_combinedTxRx_AXIMM/Combined TX and RX/Receiver HDL/Viterbi Decode ==
  validIn : Inport  SampleTime=1e-06
  reset : Inport  Port=2  SampleTime=1e-06
  crcEnd : Inport  Port=3  SampleTime=1e-06
  Bits : Inport  Port=4  PortDimensions=2  SampleTime=1e-06
  packetLenIn : Inport  Port=5  SampleTime=1e-06
  Align with post reset data : Delay  DelayLength=hex2num('3ff0000000000000')  InitialCondition=0  InputProcessing=Inherited  SampleTime=1e-06
  Buffer : Subsystem
  Logical Operator : Logic  AllPortsSameDT=off  OutDataTypeStr=boolean  SampleTime=1e-06
  Viterbi Decoder : Subsystem
  Viterbi Lag{,1..3} (4 alike) : Delay  DelayLength=hex2num('4041000000000000')  InitialCondition=0  InputProcessing=Inherited  SampleTime=1e-06
  delayMatch : Delay  DelayLength=hex2num('4034000000000000')  InitialCondition=0  InputProcessing=Inherited  SampleTime=1e-06
  validOut : Outport  InitialOutput=0
  Decoded Bits : Outport  Port=2  InitialOutput=0
  crcEndOut : Outport  Port=3  InitialOutput=0
  frameStart : Outport  Port=4  InitialOutput=0
  packetLenOut : Outport  Port=5  InitialOutput=0
  wires:
  Align with post reset data/1 -> Viterbi Lag2/1
  Buffer/1(dataOut) -> Viterbi Decoder/1(In1)
  Buffer/2(resetOut) -> Align with post reset data/1, Viterbi Decoder/2(In2)
  Buffer/3(validOut) -> Viterbi Lag/1
  Buffer/4(crcOut) -> Viterbi Lag1/1
  Buffer/5(packetLenOut) -> Viterbi Lag3/1
  Logical Operator/1 -> Decoded Bits/1
  Viterbi Decoder/1(Out1) -> Logical Operator/1
  delayMatch/1 -> Logical Operator/2
  Viterbi Lag1/1 -> crcEndOut/1
  Viterbi Lag2/1 -> frameStart/1
  Viterbi Lag3/1 -> packetLenOut/1
  validIn/1 -> Buffer/3(valid)
  reset/1 -> Buffer/2(start)
  crcEnd/1 -> Buffer/4(crc)
  Bits/1 -> Buffer/1(data)
  packetLenIn/1 -> Buffer/5(packetLen)
  Viterbi Lag/1 -> delayMatch/1, validOut/1

== system gm_combinedTxRx_AXIMM/Combined TX and RX/Transmitter HDL/DMA Interface ==
  byteIn : Inport  SampleTime=4e-06
  validIn : Inport  Port=2  SampleTime=4e-06
  EOF : Inport  Port=3  SampleTime=4e-06
  Align with data : Delay  DelayLength=1
  DMA Control : Subsystem
  validOut : Outport
  bit : Outport  Port=2
  payloadLength : Outport  Port=3  OutDataTypeStr=uint16
  startOut : Outport  Port=4
  readyForMore : Outport  Port=5
  wires:
  byteIn/1 -> DMA Control/1(byteIn)
  validIn/1 -> DMA Control/2(validIn)
  EOF/1 -> DMA Control/3(EOF)
  Align with data/1 -> startOut/1
  DMA Control/1(bitOut) -> bit/1
  DMA Control/2(validOut) -> validOut/1
  DMA Control/3(startOut) -> Align with data/1
  DMA Control/4(payloadLength) -> payloadLength/1
  DMA Control/5(readyForInput) -> readyForMore/1

== system gm_combinedTxRx_AXIMM/Combined TX and RX/Transmitter HDL/Packet Generation ==
  bits : Inport  OutDataTypeStr=boolean  SampleTime=4e-06
  payloadSize : Inport  Port=2  SampleTime=4e-06
  start : Inport  Port=3  SampleTime=4e-06
  Delay For Preamble For Preamble : Delay  DelayLength=hex2num('407a500000000000')  InitialCondition=0  InputProcessing=Inherited  SampleTime=4e-06
  Delay For Reset1 : Delay  DelayLength=hex2num('3ff0000000000000')  InitialCondition=0  InputProcessing=Inherited  SampleTime=4e-06
  Delay For Reset2 : Delay  DelayLength=hex2num('3ff0000000000000')  InitialCondition=0  InputProcessing=Inherited  SampleTime=4e-06
  Display1 : Display
  Enable Mod and Filter : simulink/Logic and Bit Operations/Compare To Constant  relop=<  const=fi(0,0,8,0,'hex','04')  OutDataTypeStr=boolean
  Frame Indexer : hdlsllib/Sources/HDL Counter  CountType=Count limited  CountInit=hex2num('0000000000000000')  CountStep=hex2num('3ff0000000000000')  CountMax=hex2num('40f01c6000000000')  CountFromType=Initial value  CountFrom=hex2num('0000000000000000')  CountResetPort=on  CountLoadPort=off  CountEnbPort=off  CountDirPort=off  CountDataType=Unsigned  CountWordLen=32  CountFracLen=0  CountSampTime=4e-06
      settings: SourceProductBaseCode=HD
  Multiport Switch : MultiPortSwitch  Inputs=4  DiagnosticForDefault=None  SampleTime=4e-06
  Multiport Switch1 : MultiPortSwitch  Inputs=4  DiagnosticForDefault=None  SampleTime=4e-06
  Payload : Subsystem
  Preamble : Subsystem
  QPSK Modulator Baseband1 : commdigbbndpm3/QPSK Modulator Baseband  InType=Bit  Enc=Binary  Ph=pi/4  outDtype=Fixed-point  outWordLen=16  outUDDataType=sfix(16)  outFracLenMode=User-defined  outFracLen=15  outDataTypeStr=fixdt(1,16,15)  outLastDataTypeStr=fixdt(1,16,15)
  Random Data : Subsystem
  Tx Controller : Subsystem
  concatenate : Concatenate
  trueData : Outport  InitialOutput=0
  symbols : Outport  Port=2  InitialOutput=complex(0)
  EOF : Outport  Port=3  OutDataTypeStr=boolean  InitialOutput=0
  wires:
  bits/1 -> Delay For Preamble For Preamble/1
  payloadSize/1 -> Tx Controller/2(payloadSize)
  start/1 -> Frame Indexer/1, Tx Controller/4(start)
  Delay For Preamble For Preamble/1 -> Delay For Reset2/1
  Delay For Reset1/1 -> Tx Controller/3(count)
  Delay For Reset2/1 -> Tx Controller/1(payloadBit)
  Frame Indexer/1 -> Delay For Reset1/1
  Multiport Switch/1 -> QPSK Modulator Baseband1/1
  Multiport Switch1/1 -> trueData/1
  Payload/1(bits) -> Multiport Switch/4
  Payload/2(end) -> EOF/1
  Payload/3(valid) -> Multiport Switch1/4
  Preamble/1(Out1) -> Multiport Switch/2
  QPSK Modulator Baseband1/1 -> symbols/1
  Random Data/1(Out1) -> Multiport Switch/5
  Tx Controller/1(modeOut) -> Multiport Switch/1, Multiport Switch1/1, Enable Mod and Filter/1, Payload/4(mode), Display1/1
  Tx Controller/2(headerData) -> concatenate/2, concatenate/1
  Tx Controller/3(data) -> Payload/1(data)
  Tx Controller/4(dataStart) -> Payload/2(start)
  Tx Controller/5(dataEnd) -> Random Data/1(In1), Payload/3(done)
  Tx Controller/6(preambleReset) -> Preamble/1(reset)
  Enable Mod and Filter/1 -> Multiport Switch1/5, Multiport Switch1/3, Multiport Switch1/2
  concatenate/1 -> Multiport Switch/3

== system gm_combinedTxRx_AXIMM/Combined TX and RX/Transmitter HDL/Raised Cosine Transmit Filter1 ==
  In1 : Inport  OutDataTypeStr=fixdt(1, 16, 15)  SampleTime=4e-06
      settings: SignalType=complex
  FIR Interpolation : dspmlti4/FIR Interpolation  FilterSource=Dialog parameters  h=filt.coeff  L=filt.rateFactor  FilterObject=Hm_firinterp  framing=Allow multirate processing  outputBufInitCond=0  roundingMode=Floor  overflowMode=off  firstCoeffDataTypeStr=Inherit: Same word length as input  firstCoeffMin=[]  firstCoeffMax=[]  firstCoeffLastDataTypeStr=Inherit: Same word length as input  outputMode=Binary point scaling  outputWordLength=hex2num('4030000000000000')  outputFracLength=hex2num('402c000000000000')  outputDataTypeStr=fixdt(1,hex2num('4030000000000000'),hex2num('402c000000000000'))  outputMin=[]  outputMax=[]  outputLastDataTypeStr=fixdt(1,hex2num('4030000000000000'),hex2num('402c000000000000'))
      settings: SourceProductName=DSP System Toolbox
  Out1 : Outport
  wires:
  In1/1 -> FIR Interpolation/1
  FIR Interpolation/1 -> Out1/1

== system gm_combinedTxRx_AXIMM/Combined TX and RX/Transmitter HDL/Subsystem ==
  In1 : Inport  SampleTime=1e-06
  Downsample5 : DownSample  N=hex2num('4010000000000000')  phase=hex2num('0000000000000000')  RateOptions=Allow multirate processing
  Sum of Elements : Sum  Inputs=+  AccumDataTypeStr=fixdt(0, 64, 0)  OutDataTypeStr=fixdt(0, 64, 0)  SampleTime=4e-06
  Tapped Delay_tap1 : Delay  DelayLength=hex2num('3ff0000000000000')  InputProcessing=Inherited  SampleTime=1e-06
  Tapped Delay_tap2 : Delay  DelayLength=hex2num('3ff0000000000000')  InputProcessing=Inherited  SampleTime=1e-06
  Tapped Delay_tap3 : Delay  DelayLength=hex2num('3ff0000000000000')  InputProcessing=Inherited  SampleTime=1e-06
  t : Mux
  Out1 : Outport
  wires:
  In1/1 -> Tapped Delay_tap1/1, t/4
  Downsample5/1 -> Sum of Elements/1
  Sum of Elements/1 -> Out1/1
  t/1 -> Downsample5/1
  Tapped Delay_tap1/1 -> Tapped Delay_tap2/1, t/3
  Tapped Delay_tap2/1 -> Tapped Delay_tap3/1, t/2
  Tapped Delay_tap3/1 -> t/1

== system gm_combinedTxRx_AXIMM/Combined TX and RX/Transmitter HDL/Subsystem1 ==
  In1 : Inport  SampleTime=1e-06
  Downsample5 : DownSample  N=hex2num('4010000000000000')  phase=hex2num('0000000000000000')  RateOptions=Allow multirate processing
  Logical Operator : Logic  Operator=OR  Inputs=1  AllPortsSameDT=off  OutDataTypeStr=boolean  SampleTime=4e-06
  Tapped Delay_tap1 : Delay  DelayLength=hex2num('3ff0000000000000')  InputProcessing=Inherited  SampleTime=1e-06
  Tapped Delay_tap2 : Delay  DelayLength=hex2num('3ff0000000000000')  InputProcessing=Inherited  SampleTime=1e-06
  Tapped Delay_tap3 : Delay  DelayLength=hex2num('3ff0000000000000')  InputProcessing=Inherited  SampleTime=1e-06
  t : Mux
  Out1 : Outport
  wires:
  In1/1 -> Tapped Delay_tap1/1, t/4
  Downsample5/1 -> Logical Operator/1
  Logical Operator/1 -> Out1/1
  t/1 -> Downsample5/1
  Tapped Delay_tap1/1 -> Tapped Delay_tap2/1, t/3
  Tapped Delay_tap2/1 -> Tapped Delay_tap3/1, t/2
  Tapped Delay_tap3/1 -> t/1

== system gm_combinedTxRx_AXIMM/Combined TX and RX/Receiver HDL/CRC Check and DMA Pack/CRC Check ES ==
  Valid : Inport  SampleTime=1e-06
  Bits : Inport  Port=2  SampleTime=1e-06
  endCRC : Inport  Port=3  SampleTime=1e-06
  StartData : Inport  Port=4  SampleTime=1e-06
  payloadLen : Inport  Port=5  SampleTime=1e-06
  CRC Decode Lag : Delay  DelayLength=hex2num('4041000000000000')  InitialCondition=0  InputProcessing=Inherited  SampleTime=1e-06
  Convert To fi : DataTypeConversion  OutDataTypeStr=fixdt(0, 1, 0)  SampleTime=1e-06  SaturateOnIntegerOverflow=on
  General CRC Syndrom Detector HDL Optimized : commcrc2/General CRC Syndrome Detector HDL Optimized  Polynomial=crc32Poly  InitialState=0  DirectMethod=off  ReflectInput=off  ReflectCRCChecksum=off  FinalXORValue=0  SimulateUsing=Code generation
      settings: SourceProductName=Communications System Toolbox  SourceProductBaseCode=CM
  delayMatch : Delay  DelayLength=hex2num('4034000000000000')  InitialCondition=0  InputProcessing=Inherited  SampleTime=1e-06
  delayMatch1 : Delay  DelayLength=hex2num('4034000000000000')  InitialCondition=0  InputProcessing=Inherited  SampleTime=1e-06
  delayMatch2 : Delay  DelayLength=hex2num('4034000000000000')  InitialCondition=0  InputProcessing=Inherited  SampleTime=1e-06
  dataOut : Outport  InitialOutput=0
  startOut : Outport  Port=2  InitialOutput=0
  endOut : Outport  Port=3  InitialOutput=0
  validOut : Outport  Port=4  InitialOutput=0
  err : Outport  Port=5  InitialOutput=0
  payloadLenOut : Outport  Port=6  InitialOutput=0
  wires:
  delayMatch2/1 -> General CRC Syndrom Detector HDL Optimized/4
  delayMatch1/1 -> General CRC Syndrom Detector HDL Optimized/3
  delayMatch/1 -> General CRC Syndrom Detector HDL Optimized/2
  CRC Decode Lag/1 -> payloadLenOut/1
  Convert To fi/1 -> General CRC Syndrom Detector HDL Optimized/1
  General CRC Syndrom Detector HDL Optimized/1 -> dataOut/1
  General CRC Syndrom Detector HDL Optimized/2 -> startOut/1
  General CRC Syndrom Detector HDL Optimized/3 -> endOut/1
  General CRC Syndrom Detector HDL Optimized/4 -> validOut/1
  General CRC Syndrom Detector HDL Optimized/5 -> err/1
  Valid/1 -> delayMatch2/1
  Bits/1 -> Convert To fi/1
  endCRC/1 -> delayMatch1/1
  StartData/1 -> delayMatch/1
  payloadLen/1 -> CRC Decode Lag/1

== system gm_combinedTxRx_AXIMM/Combined TX and RX/Receiver HDL/CRC Check and DMA Pack/DMA Interface ==
  bitIn : Inport  SampleTime=1e-06
  startIn : Inport  Port=2  SampleTime=1e-06
  endIn : Inport  Port=3  SampleTime=1e-06
  validIn : Inport  Port=4  SampleTime=1e-06
  err : Inport  Port=5  SampleTime=1e-06
  payloadLen : Inport  Port=6  SampleTime=1e-06
  Bit Packer : Subsystem
  Convert Payload Length To Bytes : Subsystem
  Data Type Conversion : DataTypeConversion  OutDataTypeStr=boolean
  Delay : Delay  DelayLength=1
  Delay Error To Last Byte of Out : Delay  DelayLength=1
  Display : Display
  byteOut : Outport
  validOut : Outport  Port=2
  sync : Outport  Port=3
  payloadLenOut : Outport  Port=4
  wires:
  Bit Packer/1(byteOut) -> Display/1, byteOut/1
  Bit Packer/2(validOut) -> validOut/1
  Bit Packer/3(startOut) -> sync/1
  Convert Payload Length To Bytes/1(packetLengthOut) -> payloadLenOut/1
  Data Type Conversion/1 -> Bit Packer/1(bitIn)
  Delay/1 -> Bit Packer/3(endIn)
  Delay Error To Last Byte of Out/1 -> Bit Packer/4(err)
  bitIn/1 -> Data Type Conversion/1
  startIn/1 -> Bit Packer/2(startIn)
  endIn/1 -> Delay/1
  validIn/1 -> Bit Packer/5(validIn)
  err/1 -> Delay Error To Last Byte of Out/1
  payloadLen/1 -> Convert Payload Length To Bytes/1(In1)
